simulink model "debug_conversion_SLOW"  (R2018b)
settings: Solver=FixedStepDiscrete  StartTime=0.0  StopTime=10.0  FixedStep=tS  RelTol=1e-3  EnableMultiTasking=on
libraries: slrtlib x2
settings Model: DataDictionary=mloc_debug_signal_conversion.sldd  Creator=ge34qer  LastModifiedBy=Admin
settings SolverCC: AutoInsertRateTranBlk=on
settings DataIOCC: SaveFormat=StructureWithTime
settings OptimizationCC: BlockReduction=off  OptimizeBlockIOStorage=off  BufferReuse=off  GlobalBufferReuse=off  ExpressionFolding=off  LocalBlockOutputs=off  OptimizeDataStoreBuffers=off  BusAssignmentInplaceUpdate=off
settings DebuggingCC: MergeDetectMultiDrivingBlocksExec=none
settings HardwareCC: ProdBitPerPointer=32  ProdBitPerSizeT=32  ProdBitPerPtrDiffT=32  ProdLargestAtomicFloat=None  ProdWordSize=32  ProdLongLongMode=on  ProdHWDeviceType=Generic->32-bit x86 compatible
settings ModelReferenceCC: ModelReferenceNumInstancesAllowed=Single  PropagateSignalLabelsOutOfModel=off
settings RTWCC: SystemTargetFile=slrt.tlc  GenCodeOnly=on  TemplateMakefile=slrt_default_tmf  Description=Simulink Real-Time  CodeExecutionProfiling=on  RTWCompilerOptimization=on
settings SimulinkRealTimeCC: SupportVariableSizeSignals=on  PreserveStateflowLocalDataDimensions=off  RL32LogTETModifier=off  xPCConcurrentTasks=on

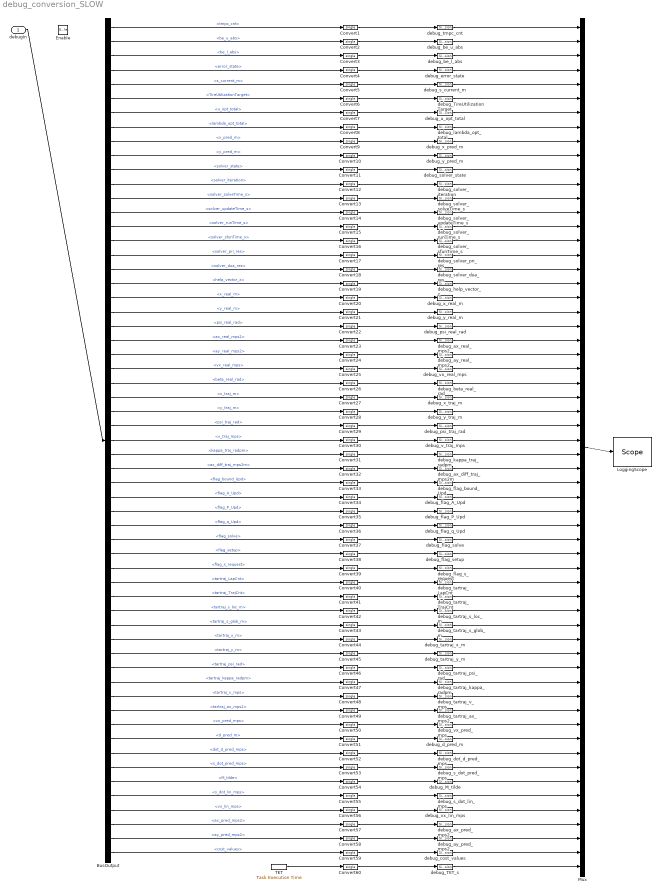
== system debug_conversion_SLOW ==
  debugIn : Inport  OutDataTypeStr=Bus: mvdc_tube_mpc_debug
  Enable : EnablePort
  BusOutput : BusSelector  OutputSignals=tmpc_cnt,be_u_abs,be_l_abs,error_state,s_current_m,TireUtilizationTarget,u_opt_total,lambda_opt_total,x_pred_m,y_pred_m,solver_state,solver_iteration,solver_solveTime_s,solver_updateTime_s,solver_runTime_s,solver_sfunTime_s,solver_pri_res,solver_dua_res,help_vector_z,x_real_m,y_real_m,psi_real_rad,ax_real_mps2,ay_real_mps2,vx_real_mps,beta_real_rad,x_traj_m,y_traj_m,psi_traj_rad,v_traj_mps,kappa_traj_radpm,ax_diff_traj_mps2m,flag_bound_Upd,flag_A_Upd,flag_P_Upd,flag_q_Upd,flag_solve,flag_setup,flag_s_request,tartraj_LapCnt,tartraj_TrajCnt,tartraj_s_loc_m,tartraj_s_glob_m,tartraj_x_m,tartraj_y_m,tartraj_psi_rad,tartraj_kappa_radpm,tartraj_v_mps,tartraj_ax_mps2,vx_pred_mps,d_pred_m,dot_d_pred_mps,s_dot_pred_mps,M_tilde,s_dot_lin_mps,vx_lin_mps,ax_pred_mps2,ay_pred_mps2,cost_values
  Convert{1..60} (60 alike) : DataTypeConversion  OutDataTypeStr=single  SaturateOnIntegerOverflow=on  RndMeth=Zero
  LoggingScope : slrtlib/Displays and Logging/Scope   scopeno=7  scopetype=File  autostart=on  viewmode=Graphical redraw  formatstr='%15.6f'  grid=on  ylimits=[0,0]  nosamples=1000  noprepostsamples=0  interleave=1  triggermode=FreeRun  triggersignal=1  trigsignalfromport=off  triggerlevel=0.0  triggerslope=Either  triggerscope=1  triggersample=0  filename=C:\LOGS\SLOW_001.dat  mode=Commit  writesize=10*512  autorestart=on  dynamicfilemode=off  maxwritefilesize=512*2048^2
  Mux : Mux  Inputs=60
  TET : slrtlib/Target Management/Execution Parameters/Task Execution Time   ts=tS
      settings: SourceProductName=Simulink Real-Time  SourceProductBaseCode=XP
  debug_M_tilde : SignalConversion  OverrideOpt=off
  debug_TET_s : SignalConversion  OverrideOpt=off
  debug_TireUtilizationTarget : SignalConversion  OverrideOpt=off
  debug_ax_diff_traj_mps2m : SignalConversion  OverrideOpt=off
  debug_ax_pred_mps2 : SignalConversion  OverrideOpt=off
  debug_ax_real_mps2 : SignalConversion  OverrideOpt=off
  debug_ay_pred_mps2 : SignalConversion  OverrideOpt=off
  debug_ay_real_mps2 : SignalConversion  OverrideOpt=off
  debug_be_l_abs : SignalConversion  OverrideOpt=off
  debug_be_u_abs : SignalConversion  OverrideOpt=off
  debug_beta_real_rad : SignalConversion  OverrideOpt=off
  debug_cost_values : SignalConversion  OverrideOpt=off
  debug_d_pred_m : SignalConversion  OverrideOpt=off
  debug_dot_d_pred_mps : SignalConversion  OverrideOpt=off
  debug_error_state : SignalConversion  OverrideOpt=off
  debug_flag_A_Upd : SignalConversion  OverrideOpt=off
  debug_flag_P_Upd : SignalConversion  OverrideOpt=off
  debug_flag_bound_Upd : SignalConversion  OverrideOpt=off
  debug_flag_q_Upd : SignalConversion  OverrideOpt=off
  debug_flag_s_request : SignalConversion  OverrideOpt=off
  debug_flag_setup : SignalConversion  OverrideOpt=off
  debug_flag_solve : SignalConversion  OverrideOpt=off
  debug_help_vector_z : SignalConversion  OverrideOpt=off
  debug_kappa_traj_radpm : SignalConversion  OverrideOpt=off
  debug_lambda_opt_total : SignalConversion  OverrideOpt=off
  debug_psi_real_rad : SignalConversion  OverrideOpt=off
  debug_psi_traj_rad : SignalConversion  OverrideOpt=off
  debug_s_current_m : SignalConversion  OverrideOpt=off
  debug_s_dot_lin_mps : SignalConversion  OverrideOpt=off
  debug_s_dot_pred_mps : SignalConversion  OverrideOpt=off
  debug_solver_dua_res : SignalConversion  OverrideOpt=off
  debug_solver_iteration : SignalConversion  OverrideOpt=off
  debug_solver_pri_res : SignalConversion  OverrideOpt=off
  debug_solver_runTime_s : SignalConversion  OverrideOpt=off
  debug_solver_sfunTime_s : SignalConversion  OverrideOpt=off
  debug_solver_solveTime_s : SignalConversion  OverrideOpt=off
  debug_solver_state : SignalConversion  OverrideOpt=off
  debug_solver_updateTime_s : SignalConversion  OverrideOpt=off
  debug_tartraj_LapCnt : SignalConversion  OverrideOpt=off
  debug_tartraj_TrajCnt : SignalConversion  OverrideOpt=off
  debug_tartraj_ax_mps2 : SignalConversion  OverrideOpt=off
  debug_tartraj_kappa_radpm : SignalConversion  OverrideOpt=off
  debug_tartraj_psi_rad : SignalConversion  OverrideOpt=off
  debug_tartraj_s_glob_m : SignalConversion  OverrideOpt=off
  debug_tartraj_s_loc_m : SignalConversion  OverrideOpt=off
  debug_tartraj_v_mps : SignalConversion  OverrideOpt=off
  debug_tartraj_x_m : SignalConversion  OverrideOpt=off
  debug_tartraj_y_m : SignalConversion  OverrideOpt=off
  debug_tmpc_cnt : SignalConversion  OverrideOpt=off
  debug_u_opt_total : SignalConversion  OverrideOpt=off
  debug_v_traj_mps : SignalConversion  OverrideOpt=off
  debug_vx_lin_mps : SignalConversion  OverrideOpt=off
  debug_vx_pred_mps : SignalConversion  OverrideOpt=off
  debug_vx_real_mps : SignalConversion  OverrideOpt=off
  debug_x_pred_m : SignalConversion  OverrideOpt=off
  debug_x_real_m : SignalConversion  OverrideOpt=off
  debug_x_traj_m : SignalConversion  OverrideOpt=off
  debug_y_pred_m : SignalConversion  OverrideOpt=off
  debug_y_real_m : SignalConversion  OverrideOpt=off
  debug_y_traj_m : SignalConversion  OverrideOpt=off
  wires:
  debugIn/1 -> BusOutput/1
  Convert1/1 -> debug_tmpc_cnt/1
  BusOutput/1 -> Convert1/1  "<tmpc_cnt>"
  debug_tmpc_cnt/1 -> Mux/1
  Convert2/1 -> debug_be_u_abs/1
  BusOutput/2 -> Convert2/1  "<be_u_abs>"
  debug_be_u_abs/1 -> Mux/2
  Convert3/1 -> debug_be_l_abs/1
  BusOutput/3 -> Convert3/1  "<be_l_abs>"
  debug_be_l_abs/1 -> Mux/3
  Convert4/1 -> debug_error_state/1
  BusOutput/4 -> Convert4/1  "<error_state>"
  debug_error_state/1 -> Mux/4
  Convert5/1 -> debug_s_current_m/1
  BusOutput/5 -> Convert5/1  "<s_current_m>"
  debug_s_current_m/1 -> Mux/5
  Convert6/1 -> debug_TireUtilizationTarget/1
  BusOutput/6 -> Convert6/1  "<TireUtilizationTarget>"
  debug_TireUtilizationTarget/1 -> Mux/6
  Convert7/1 -> debug_u_opt_total/1
  BusOutput/7 -> Convert7/1  "<u_opt_total>"
  debug_u_opt_total/1 -> Mux/7
  Convert8/1 -> debug_lambda_opt_total/1
  BusOutput/8 -> Convert8/1  "<lambda_opt_total>"
  debug_lambda_opt_total/1 -> Mux/8
  Convert9/1 -> debug_x_pred_m/1
  BusOutput/9 -> Convert9/1  "<x_pred_m>"
  debug_x_pred_m/1 -> Mux/9
  Convert10/1 -> debug_y_pred_m/1
  BusOutput/10 -> Convert10/1  "<y_pred_m>"
  debug_y_pred_m/1 -> Mux/10
  Convert11/1 -> debug_solver_state/1
  BusOutput/11 -> Convert11/1  "<solver_state>"
  debug_solver_state/1 -> Mux/11
  Convert12/1 -> debug_solver_iteration/1
  BusOutput/12 -> Convert12/1  "<solver_iteration>"
  debug_solver_iteration/1 -> Mux/12
  Convert13/1 -> debug_solver_solveTime_s/1
  BusOutput/13 -> Convert13/1  "<solver_solveTime_s>"
  debug_solver_solveTime_s/1 -> Mux/13
  Convert14/1 -> debug_solver_updateTime_s/1
  BusOutput/14 -> Convert14/1  "<solver_updateTime_s>"
  debug_solver_updateTime_s/1 -> Mux/14
  Convert15/1 -> debug_solver_runTime_s/1
  BusOutput/15 -> Convert15/1  "<solver_runTime_s>"
  debug_solver_runTime_s/1 -> Mux/15
  Convert16/1 -> debug_solver_sfunTime_s/1
  BusOutput/16 -> Convert16/1  "<solver_sfunTime_s>"
  debug_solver_sfunTime_s/1 -> Mux/16
  Convert17/1 -> debug_solver_pri_res/1
  BusOutput/17 -> Convert17/1  "<solver_pri_res>"
  debug_solver_pri_res/1 -> Mux/17
  Convert18/1 -> debug_solver_dua_res/1
  BusOutput/18 -> Convert18/1  "<solver_dua_res>"
  debug_solver_dua_res/1 -> Mux/18
  Convert19/1 -> debug_help_vector_z/1
  BusOutput/19 -> Convert19/1  "<help_vector_z>"
  debug_help_vector_z/1 -> Mux/19
  Convert20/1 -> debug_x_real_m/1
  BusOutput/20 -> Convert20/1  "<x_real_m>"
  debug_x_real_m/1 -> Mux/20
  Convert21/1 -> debug_y_real_m/1
  BusOutput/21 -> Convert21/1  "<y_real_m>"
  debug_y_real_m/1 -> Mux/21
  Convert22/1 -> debug_psi_real_rad/1
  BusOutput/22 -> Convert22/1  "<psi_real_rad>"
  debug_psi_real_rad/1 -> Mux/22
  Convert23/1 -> debug_ax_real_mps2/1
  BusOutput/23 -> Convert23/1  "<ax_real_mps2>"
  debug_ax_real_mps2/1 -> Mux/23
  Convert24/1 -> debug_ay_real_mps2/1
  BusOutput/24 -> Convert24/1  "<ay_real_mps2>"
  debug_ay_real_mps2/1 -> Mux/24
  Convert25/1 -> debug_vx_real_mps/1
  BusOutput/25 -> Convert25/1  "<vx_real_mps>"
  debug_vx_real_mps/1 -> Mux/25
  Convert26/1 -> debug_beta_real_rad/1
  BusOutput/26 -> Convert26/1  "<beta_real_rad>"
  debug_beta_real_rad/1 -> Mux/26
  Convert27/1 -> debug_x_traj_m/1
  BusOutput/27 -> Convert27/1  "<x_traj_m>"
  debug_x_traj_m/1 -> Mux/27
  Convert28/1 -> debug_y_traj_m/1
  BusOutput/28 -> Convert28/1  "<y_traj_m>"
  debug_y_traj_m/1 -> Mux/28
  Convert29/1 -> debug_psi_traj_rad/1
  BusOutput/29 -> Convert29/1  "<psi_traj_rad>"
  debug_psi_traj_rad/1 -> Mux/29
  Convert30/1 -> debug_v_traj_mps/1
  BusOutput/30 -> Convert30/1  "<v_traj_mps>"
  debug_v_traj_mps/1 -> Mux/30
  Convert31/1 -> debug_kappa_traj_radpm/1
  BusOutput/31 -> Convert31/1  "<kappa_traj_radpm>"
  debug_kappa_traj_radpm/1 -> Mux/31
  Convert32/1 -> debug_ax_diff_traj_mps2m/1
  BusOutput/32 -> Convert32/1  "<ax_diff_traj_mps2m>"
  debug_ax_diff_traj_mps2m/1 -> Mux/32
  Convert33/1 -> debug_flag_bound_Upd/1
  BusOutput/33 -> Convert33/1  "<flag_bound_Upd>"
  debug_flag_bound_Upd/1 -> Mux/33
  Convert34/1 -> debug_flag_A_Upd/1
  BusOutput/34 -> Convert34/1  "<flag_A_Upd>"
  debug_flag_A_Upd/1 -> Mux/34
  Convert35/1 -> debug_flag_P_Upd/1
  BusOutput/35 -> Convert35/1  "<flag_P_Upd>"
  debug_flag_P_Upd/1 -> Mux/35
  Convert36/1 -> debug_flag_q_Upd/1
  BusOutput/36 -> Convert36/1  "<flag_q_Upd>"
  debug_flag_q_Upd/1 -> Mux/36
  Convert37/1 -> debug_flag_solve/1
  BusOutput/37 -> Convert37/1  "<flag_solve>"
  debug_flag_solve/1 -> Mux/37
  Convert38/1 -> debug_flag_setup/1
  BusOutput/38 -> Convert38/1  "<flag_setup>"
  debug_flag_setup/1 -> Mux/38
  Convert39/1 -> debug_flag_s_request/1
  BusOutput/39 -> Convert39/1  "<flag_s_request>"
  debug_flag_s_request/1 -> Mux/39
  Convert40/1 -> debug_tartraj_LapCnt/1
  BusOutput/40 -> Convert40/1  "<tartraj_LapCnt>"
  debug_tartraj_LapCnt/1 -> Mux/40
  Convert41/1 -> debug_tartraj_TrajCnt/1
  BusOutput/41 -> Convert41/1  "<tartraj_TrajCnt>"
  debug_tartraj_TrajCnt/1 -> Mux/41
  Convert42/1 -> debug_tartraj_s_loc_m/1
  BusOutput/42 -> Convert42/1  "<tartraj_s_loc_m>"
  debug_tartraj_s_loc_m/1 -> Mux/42
  Convert43/1 -> debug_tartraj_s_glob_m/1
  BusOutput/43 -> Convert43/1  "<tartraj_s_glob_m>"
  debug_tartraj_s_glob_m/1 -> Mux/43
  Convert44/1 -> debug_tartraj_x_m/1
  BusOutput/44 -> Convert44/1  "<tartraj_x_m>"
  debug_tartraj_x_m/1 -> Mux/44
  Convert45/1 -> debug_tartraj_y_m/1
  BusOutput/45 -> Convert45/1  "<tartraj_y_m>"
  debug_tartraj_y_m/1 -> Mux/45
  Convert46/1 -> debug_tartraj_psi_rad/1
  BusOutput/46 -> Convert46/1  "<tartraj_psi_rad>"
  debug_tartraj_psi_rad/1 -> Mux/46
  Convert47/1 -> debug_tartraj_kappa_radpm/1
  BusOutput/47 -> Convert47/1  "<tartraj_kappa_radpm>"
  debug_tartraj_kappa_radpm/1 -> Mux/47
  Convert48/1 -> debug_tartraj_v_mps/1
  BusOutput/48 -> Convert48/1  "<tartraj_v_mps>"
  debug_tartraj_v_mps/1 -> Mux/48
  Convert49/1 -> debug_tartraj_ax_mps2/1
  BusOutput/49 -> Convert49/1  "<tartraj_ax_mps2>"
  debug_tartraj_ax_mps2/1 -> Mux/49
  Convert50/1 -> debug_vx_pred_mps/1
  BusOutput/50 -> Convert50/1  "<vx_pred_mps>"
  debug_vx_pred_mps/1 -> Mux/50
  Convert51/1 -> debug_d_pred_m/1
  BusOutput/51 -> Convert51/1  "<d_pred_m>"
  debug_d_pred_m/1 -> Mux/51
  Convert52/1 -> debug_dot_d_pred_mps/1
  BusOutput/52 -> Convert52/1  "<dot_d_pred_mps>"
  debug_dot_d_pred_mps/1 -> Mux/52
  Convert53/1 -> debug_s_dot_pred_mps/1
  BusOutput/53 -> Convert53/1  "<s_dot_pred_mps>"
  debug_s_dot_pred_mps/1 -> Mux/53
  Convert54/1 -> debug_M_tilde/1
  BusOutput/54 -> Convert54/1  "<M_tilde>"
  debug_M_tilde/1 -> Mux/54
  Convert55/1 -> debug_s_dot_lin_mps/1
  BusOutput/55 -> Convert55/1  "<s_dot_lin_mps>"
  debug_s_dot_lin_mps/1 -> Mux/55
  Convert56/1 -> debug_vx_lin_mps/1
  BusOutput/56 -> Convert56/1  "<vx_lin_mps>"
  debug_vx_lin_mps/1 -> Mux/56
  Convert57/1 -> debug_ax_pred_mps2/1
  BusOutput/57 -> Convert57/1  "<ax_pred_mps2>"
  debug_ax_pred_mps2/1 -> Mux/57
  Convert58/1 -> debug_ay_pred_mps2/1
  BusOutput/58 -> Convert58/1  "<ay_pred_mps2>"
  debug_ay_pred_mps2/1 -> Mux/58
  Convert59/1 -> debug_cost_values/1
  BusOutput/59 -> Convert59/1  "<cost_values>"
  debug_cost_values/1 -> Mux/59
  Convert60/1 -> debug_TET_s/1
  debug_TET_s/1 -> Mux/60
  TET/1 -> Convert60/1
  Mux/1 -> LoggingScope/1
